simulink model "Wind_Turbine"  (R2018a)
settings: Solver=ode3  StartTime=0.0  StopTime=80  FixedStep=1e-4  RelTol=1e-3  EnableMultiTasking=on
InitFcn:
  | clear all ;
  | clc;
  | %Turbine
  | R_=45;
  | G=100;
  | lambda_opt=7.07;
  | Rho=1.225;
  | J=254;
  | f=0.01;
  | 
  | %RL filter;
  | 
  | fs=10000;
  | fe=50;
  | Ws=2*pi*fe;
  | Pres=3e6;
  | L=0.75e-3;
  | R=0.075;
  | c=38e-3;
  | 
  | %Commande CCR;
  | 
  | Id_=300;
  | Vdc_=1200;
  | %Vq_=0;
  | tr=0.001;
  | kp=3*L/tr;
  | ki=3*R/tr;
  | 
  | %CCM Commande;
  | 
  | p=2;p=2;
  | Tr=0.02;
  | Lfs=121e-6;
  | Lfr=57.3e-6;
  | Lm=12.12e-3;
  | m=1;
  | Ls=Lfs+Lm;
  | Lr=Lfr+m*Lm;
  | sigma=1-(m*Lm)^2/(Ls*Lr);
  | Rr=3.82e-3;
  | Rs=2.97e-3;
  | kpr=3*sigma*Lr/Tr;
  | kir=3*Rr/Tr;
  | Qs_ref=0;
undefined symbols (not defined in the file): sigbuilder_block
libraries: powerlib_meascontrol x8, simulink x4
settings Model: Creator=PC  LastModifiedBy=yassine
settings OptimizationCC: LifeSpan=inf
settings DebuggingCC: SFUnexpectedBacktrackingDiag=warning  SFNoUnconditionalDefaultTransitionDiag=warning
settings CodeAppCC: StateflowObjectComments=on
settings GRTTargetCC: TargetLangStandard=C89/C90 (ANSI)
settings ConfigComp: CovMetricSettings=dw  CovSaveCumulativeToWorkspaceVar=on  CovSaveSingleToWorkspaceVar=on  CovExternalEMLEnable=off

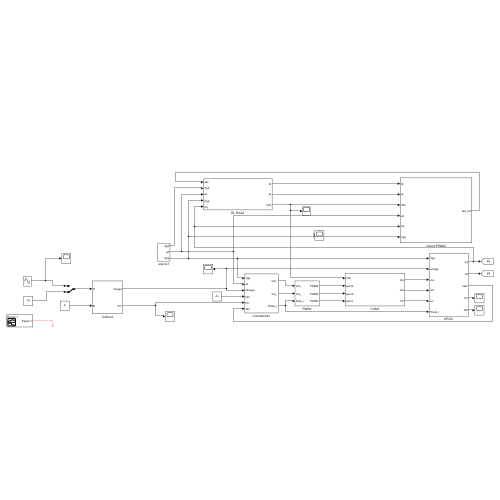
[thumbnail: Simulink's stored preview of the top-level diagram]
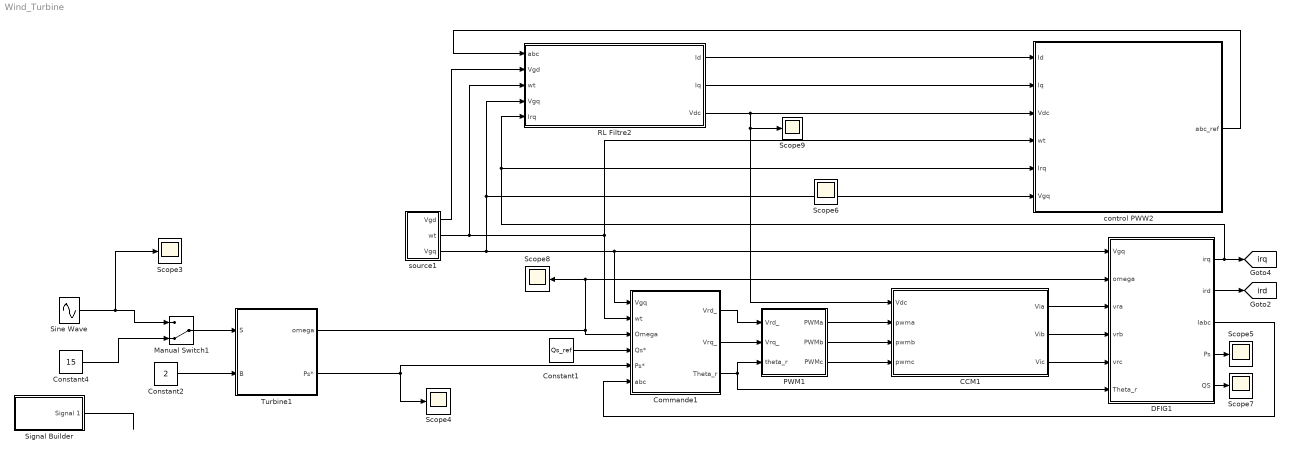
== system Wind_Turbine ==
  CCM1 : Subsystem
  Commande1 : Subsystem
  Constant1 : Constant  Value=Qs_ref
  Constant2 : Constant  Value=2
  Constant4 : Constant  Value=15
  DFIG1 : Subsystem
  Manual Switch1 : ManualSwitch  CurrentSetting=0
  PWM1 : Subsystem
  RL Filtre2 : Subsystem  InitFcn=""
  Scope{3..9} (7 alike) : Scope
  Signal Builder : Subsystem  Tag=STV Subsys  LoadFcn=sigbuilder_block('load');  StartFcn=sigbuilder_block('start');  StopFcn=sigbuilder_block('stop');  ClipboardFcn=sigbuilder_block('clipboard');  mask(Sigbuilder block){tuvar=[0:10]}
      mask help: Simulink:masks:SigbuilderBlock_MD
      mask init:
      | if ~strcmp(get_param(bdroot(gcbh),'SimulationStatus'),'stopped') tuvar = sigbuilder_block('maskInit'); end
      settings: CopyFcn=sigbuilder_block('copy');  DeleteFcn=sigbuilder_block('delete');  ModelCloseFcn=sigbuilder_block('modelClose');  PreSaveFcn=sigbuilder_block('preSave');  PauseFcn=sigbuilder_block('pause');  ContinueFcn=sigbuilder_block('continue');  NameChangeFcn=sigbuilder_block('namechange');  OpenFcn=sigbuilder_block('open',[525.6 43.2 550.8 400.2 ]);  CloseFcn=sigbuilder_block('close');
      mask Display: plot(0, 0, 100, 100,[2, 2, 32, 32, 2], [68, 8, 8, 68, 68],[32, 2], [38, 38], [32, 19, 2],[53, 60, 44], [32, 17, 17, 2],[16, 16, 31, 31]);txt = getActiveGroup(gcbh);text(2, 100, txt,'verticalAlignment', 'top');
  Sine Wave : Sin  Bias=9  Frequency=2*pi*1/80  SampleTime=0
  Turbine1 : Subsystem
  control PWW2 : Subsystem
  source1 : Subsystem
  tag scope: ird=global, irq=global
  wires:
  source1/2(wt) -> Commande1/2(wt), control PWW2/4(wt), RL Filtre2/3(wt)
  CCM1/1(Via) -> DFIG1/3(vra)
  CCM1/2(Vib) -> DFIG1/4(vrb)
  CCM1/3(Vic) -> DFIG1/5(vrc)
  RL Filtre2/3(Vdc) -> CCM1/1(Vdc), Scope9/1, control PWW2/3(Vdc)
  PWM1/2(PWMb) -> CCM1/3(pwmb)
  Commande1/1(Vrd_) -> PWM1/1(Vrd_)
  Commande1/2(Vrq_) -> PWM1/2(Vrq_)
  PWM1/1(PWMa) -> CCM1/2(pwma)
  PWM1/3(PWMc) -> CCM1/4(pwmc)
  source1/3(Vgq) -> Commande1/1(Vgq), DFIG1/1(Vgq), control PWW2/6(Vgq), RL Filtre2/4(Vgq)
  Commande1/3(Theta_r) -> DFIG1/6(Theta_r), PWM1/3(theta_r)
  DFIG1/3(Iabc) -> Commande1/6(abc)
  DFIG1/2(ird) -> [ird]
  Turbine1/1(omega) -> Scope8/1, DFIG1/2(omega), Commande1/3(Omega)
  DFIG1/4(Ps) -> Scope5/1
  DFIG1/5(QS) -> Scope7/1
  control PWW2/1(abc_ref) -> RL Filtre2/1(abc)
  RL Filtre2/1(Id) -> control PWW2/1(Id)
  RL Filtre2/2(Iq) -> control PWW2/2(Iq)
  DFIG1/1(irq) -> [irq], RL Filtre2/5(Irq), control PWW2/5(Irq)
  source1/1(Vgd) -> RL Filtre2/2(Vgd)
  Constant1/1 -> Commande1/4(Qs*)
  Turbine1/2(Ps*) -> Commande1/5(Ps*), Scope4/1
  Constant2/1 -> Turbine1/2(B)
  Sine Wave/1 -> Manual Switch1/1, Scope3/1
  Manual Switch1/1 -> Turbine1/1(S)
  Signal Builder/1(Signal 1) -> ?
  Constant4/1 -> Manual Switch1/2

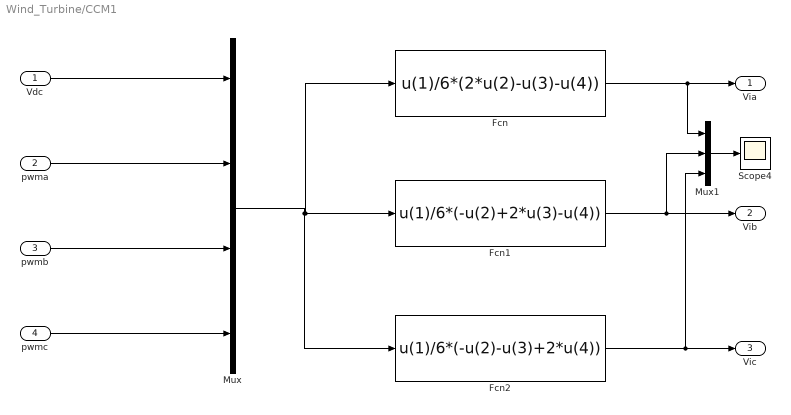
== system Wind_Turbine/CCM1 ==
  Vdc : Inport
  pwma : Inport  Port=2
  pwmb : Inport  Port=3
  pwmc : Inport  Port=4
  Fcn : Fcn  Expr=u(1)/6*(2*u(2)-u(3)-u(4))
  Fcn1 : Fcn  Expr=u(1)/6*(-u(2)+2*u(3)-u(4))
  Fcn2 : Fcn  Expr=u(1)/6*(-u(2)-u(3)+2*u(4))
  Mux : Mux
  Mux1 : Mux  Inputs=3
  Scope4 : Scope
  Via : Outport
  Vib : Outport  Port=2
  Vic : Outport  Port=3
  wires:
  Vdc/1 -> Mux/1
  Mux/1 -> Fcn2/1, Fcn1/1, Fcn/1
  pwma/1 -> Mux/2
  pwmb/1 -> Mux/3
  pwmc/1 -> Mux/4
  Fcn/1 -> Mux1/1, Via/1
  Fcn1/1 -> Vib/1, Mux1/2
  Fcn2/1 -> Vic/1, Mux1/3
  Mux1/1 -> Scope4/1

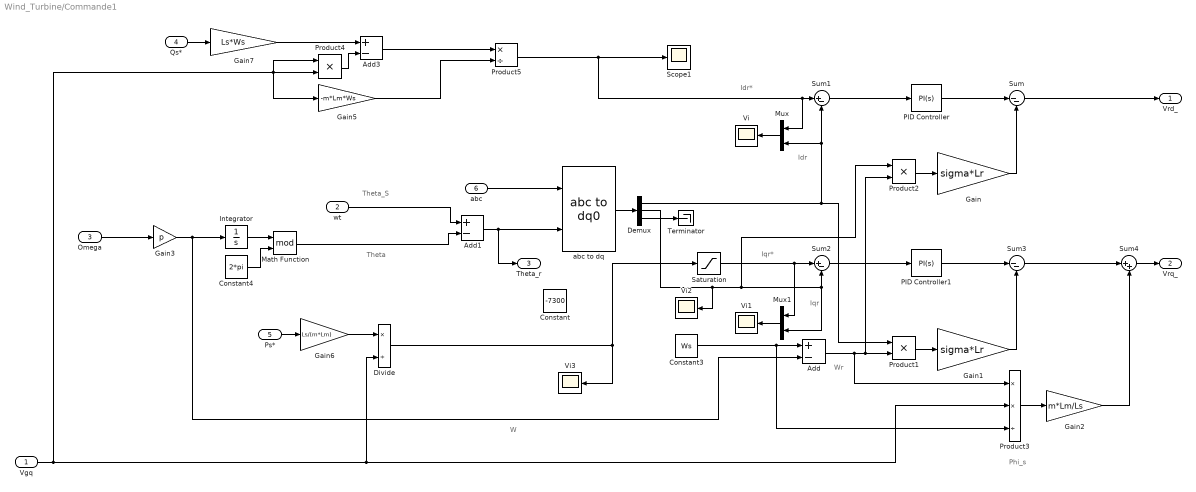
== system Wind_Turbine/Commande1 ==
  note: Theta_S
  note: Theta
  note: W
  note: Wr
  note: Iqr
  note: Idr
  note: Phi_s
  note: Idr*
  note: Iqr*
  Vgq : Inport
  wt : Inport  Port=2
  Omega : Inport  Port=3
  Qs* : Inport  Port=4
  Ps* : Inport  Port=5
  abc : Inport  Port=6
  Add : Sum  Inputs=+-
  Add1 : Sum  Inputs=+-
  Add3 : Sum  Inputs=+-
  Constant : Constant  Value=-7300
  Constant3 : Constant  Value=Ws
  Constant4 : Constant  Value=2*pi
  Demux : Demux  Outputs=3
  Divide : Product  Inputs=*/
  Gain : Gain  Gain=sigma*Lr
  Gain1 : Gain  Gain=sigma*Lr
  Gain2 : Gain  Gain=m*Lm/Ls
  Gain3 : Gain  Gain=p
  Gain5 : Gain  Gain=-m*Lm*Ws
  Gain6 : Gain  Gain=Ls/(m*Lm)
  Gain7 : Gain  Gain=Ls*Ws
  Integrator : Integrator
  Math Function : Math  Operator=mod  SaturateOnIntegerOverflow=on
  Mux : Mux  Inputs=2
  Mux1 : Mux  Inputs=2
  PID Controller : simulink/Continuous/PID Controller  Controller=PI  Form=Parallel  TimeDomain=Continuous-time  SampleTime=-1  IntegratorMethod=Forward Euler  ControllerParametersSource=internal  P=kpr*62  I=kir*62  D=0  N=100  UseFilter=on  TunerSelectOption=Transfer Function Based (PID Tuner App)  InitialConditionSource=internal  InitialConditionForIntegrator=0  InitialConditionForFilter=0  DifferentiatorICPrevScaledInput=0  ExternalReset=none  TrackingMode=off  Kt=1  LimitOutput=off  UpperSaturationLimit=inf  LowerSaturationLimit=-inf  LinearizeAsGain=on  AntiWindupMode=none  Kb=1  POutMin=[]  POutMax=[]  IOutMin=[]  IOutMax=[]  DOutMin=[]  DOutMax=[]  NOutMin=[]  NOutMax=[]  SumOutMin=[]  SumOutMax=[]  SaturationOutMin=[]  SaturationOutMax=[]  PParamMin=[]  PParamMax=[]  IParamMin=[]  IParamMax=[]  DParamMin=[]  DParamMax=[]  NParamMin=[]  NParamMax=[]  KbParamMin=[]  KbParamMax=[]  KtParamMin=[]  KtParamMax=[]  KbOutMin=[]  KbOutMax=[]  KtOutMin=[]  KtOutMax=[]  IntegratorOutMin=[]  IntegratorOutMax=[]  FilterOutMin=[]  FilterOutMax=[]  SumI1OutMin=[]  SumI1OutMax=[]  SumI2OutMin=[]  SumI2OutMax=[]  SumI3OutMin=[]  SumI3OutMax=[]  SumDOutMin=[]  SumDOutMax=[]  DifferentiatorOutMin=[]  DifferentiatorOutMax=[]  FilterDiffOutCoefMin=[]  FilterDiffOutCoefMax=[]  ReciprocalOutMin=[]  ReciprocalOutMax=[]  SumDenOutMin=[]  SumDenOutMax=[]  SumNumOutMin=[]  SumNumOutMax=[]  DivideOutMin=[]  DivideOutMax=[]  IntegratorContinuousStateAttributes=''  IntegratorStateMustResolveToSignalObject=off  IntegratorRTWStateStorageClass=Auto  FilterContinuousStateAttributes=''  FilterStateMustResolveToSignalObject=off  FilterRTWStateStorageClass=Auto
  PID Controller1 : simulink/Continuous/PID Controller  Controller=PI  Form=Parallel  TimeDomain=Continuous-time  SampleTime=-1  IntegratorMethod=Forward Euler  ControllerParametersSource=internal  P=kpr*62  I=kir*62  D=0  N=100  UseFilter=on  TunerSelectOption=Transfer Function Based (PID Tuner App)  InitialConditionSource=internal  InitialConditionForIntegrator=0  InitialConditionForFilter=0  DifferentiatorICPrevScaledInput=0  ExternalReset=none  TrackingMode=off  Kt=1  LimitOutput=off  UpperSaturationLimit=inf  LowerSaturationLimit=-inf  LinearizeAsGain=on  AntiWindupMode=none  Kb=1  POutMin=[]  POutMax=[]  IOutMin=[]  IOutMax=[]  DOutMin=[]  DOutMax=[]  NOutMin=[]  NOutMax=[]  SumOutMin=[]  SumOutMax=[]  SaturationOutMin=[]  SaturationOutMax=[]  PParamMin=[]  PParamMax=[]  IParamMin=[]  IParamMax=[]  DParamMin=[]  DParamMax=[]  NParamMin=[]  NParamMax=[]  KbParamMin=[]  KbParamMax=[]  KtParamMin=[]  KtParamMax=[]  KbOutMin=[]  KbOutMax=[]  KtOutMin=[]  KtOutMax=[]  IntegratorOutMin=[]  IntegratorOutMax=[]  FilterOutMin=[]  FilterOutMax=[]  SumI1OutMin=[]  SumI1OutMax=[]  SumI2OutMin=[]  SumI2OutMax=[]  SumI3OutMin=[]  SumI3OutMax=[]  SumDOutMin=[]  SumDOutMax=[]  DifferentiatorOutMin=[]  DifferentiatorOutMax=[]  FilterDiffOutCoefMin=[]  FilterDiffOutCoefMax=[]  ReciprocalOutMin=[]  ReciprocalOutMax=[]  SumDenOutMin=[]  SumDenOutMax=[]  SumNumOutMin=[]  SumNumOutMax=[]  DivideOutMin=[]  DivideOutMax=[]  IntegratorContinuousStateAttributes=''  IntegratorStateMustResolveToSignalObject=off  IntegratorRTWStateStorageClass=Auto  FilterContinuousStateAttributes=''  FilterStateMustResolveToSignalObject=off  FilterRTWStateStorageClass=Auto
  Product1 : Product
  Product2 : Product
  Product3 : Product  Inputs=**/
  Product4 : Product  Inputs=**
  Product5 : Product  Inputs=*/
  Saturation : Saturate  UpperLimit=8e3  LowerLimit=-8e3
  Scope1 : Scope
  Sum : Sum  Inputs=|--
  Sum1 : Sum  Inputs=|+-
  Sum2 : Sum  Inputs=|+-
  Sum3 : Sum  Inputs=|--
  Sum4 : Sum  Inputs=|++
  Terminator : Terminator
  Vi{,1..3} (4 alike) : Scope
  abc to dq : powerlib_meascontrol/Transformations/abc to dq0  Alignment=90 degrees behind phase A axis
  Vrd_ : Outport
  Vrq_ : Outport  Port=2
  Theta_r : Outport  Port=3
  wires:
  Sum2/1 -> PID Controller1/1
  Sum1/1 -> PID Controller/1
  Demux/2 -> Vi2/1, Mux1/2, Sum2/2, Product2/1
  PID Controller/1 -> Sum/1
  Gain/1 -> Sum/2
  Sum4/1 -> Vrq_/1
  PID Controller1/1 -> Sum3/1
  Demux/1 -> Sum1/2, Mux/2, Product1/1
  Gain2/1 -> Sum4/2
  Sum3/1 -> Sum4/1
  Sum/1 -> Vrd_/1
  Gain1/1 -> Sum3/2
  Constant3/1 -> Product3/3, Add/1
  Product1/1 -> Gain1/1
  Add/1 -> Product3/1, Product2/2, Product1/2
  Omega/1 -> Gain3/1
  Product2/1 -> Gain/1
  Product3/1 -> Gain2/1
  abc to dq/1 -> Demux/1
  Demux/3 -> Terminator/1
  abc/1 -> abc to dq/1
  wt/1 -> Add1/1
  Integrator/1 -> Math Function/1
  Constant4/1 -> Math Function/2
  Math Function/1 -> Add1/2
  Gain3/1 -> Integrator/1, Add/2
  Mux/1 -> Vi/1
  Mux1/1 -> Vi1/1
  Add1/1 -> abc to dq/2, Theta_r/1
  Add3/1 -> Product5/1
  Vgq/1 -> Product3/2, Divide/2, Product4/1, Gain5/1, Product4/2
  Qs*/1 -> Gain7/1
  Gain5/1 -> Product5/2
  Product5/1 -> Sum1/1, Mux/1, Scope1/1
  Ps*/1 -> Gain6/1
  Gain6/1 -> Divide/1
  Gain7/1 -> Add3/1
  Product4/1 -> Add3/2
  Divide/1 -> Vi3/1, Saturation/1
  Saturation/1 -> Mux1/1, Sum2/1

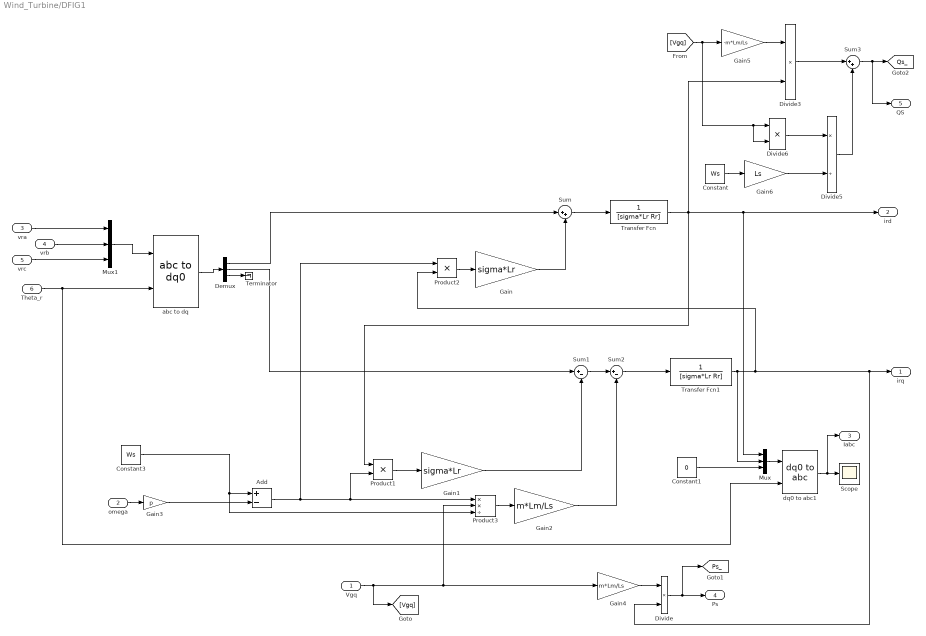
== system Wind_Turbine/DFIG1 ==
  Vgq : Inport
  omega : Inport  Port=2
  vra : Inport  Port=3
  vrb : Inport  Port=4
  vrc : Inport  Port=5
  Theta_r : Inport  Port=6
  Add : Sum  Inputs=+-
  Constant : Constant  Value=Ws
  Constant1 : Constant  Value=0
  Constant3 : Constant  Value=Ws
  Demux : Demux  Outputs=3
  Divide : Product  Inputs=**
  Divide3 : Product  Inputs=**
  Divide5 : Product  Inputs=*/
  Divide6 : Product  Inputs=**
  Gain : Gain  Gain=sigma*Lr
  Gain1 : Gain  Gain=sigma*Lr
  Gain2 : Gain  Gain=m*Lm/Ls
  Gain3 : Gain  Gain=p
  Gain4 : Gain  Gain=m*Lm/Ls
  Gain5 : Gain  Gain=-m*Lm/Ls
  Gain6 : Gain  Gain=Ls
  Mux : Mux  Inputs=3
  Mux1 : Mux  Inputs=3
  Product1 : Product
  Product2 : Product
  Product3 : Product  Inputs=**/
  Scope : Scope
  Sum : Sum  Inputs=|++
  Sum1 : Sum  Inputs=|+-
  Sum2 : Sum  Inputs=|+-
  Sum3 : Sum  Inputs=|++
  Terminator : Terminator
  Transfer Fcn : TransferFcn  Denominator=[sigma*Lr Rr]
  Transfer Fcn1 : TransferFcn  Denominator=[sigma*Lr Rr]
  abc to dq : powerlib_meascontrol/Transformations/abc to dq0  Alignment=90 degrees behind phase A axis
  dq0 to abc1 : powerlib_meascontrol/Transformations/dq0 to abc  Alignment=90 degrees behind phase A axis
  irq : Outport
  ird : Outport  Port=2
  Iabc : Outport  Port=3
  Ps : Outport  Port=4
  QS : Outport  Port=5
  tag scope: Ps_=global, Qs_=global
  wires:
  Transfer Fcn/1 -> ird/1, Mux/1, Divide3/2, Product1/1
  Sum/1 -> Transfer Fcn/1
  Demux/2 -> Sum1/1
  Demux/1 -> Sum/1
  Product2/1 -> Gain/1
  Gain/1 -> Sum/2
  Constant3/1 -> Product3/3, Add/1
  Product1/1 -> Gain1/1
  Product3/1 -> Gain2/1
  Sum1/1 -> Sum2/1
  Gain1/1 -> Sum1/2
  Gain2/1 -> Sum2/2
  Sum2/1 -> Transfer Fcn1/1
  Add/1 -> Product2/1, Product1/2, Product3/1
  omega/1 -> Gain3/1
  Gain3/1 -> Add/2
  Constant1/1 -> Mux/3
  Mux/1 -> dq0 to abc1/1
  dq0 to abc1/1 -> Iabc/1, Scope/1
  abc to dq/1 -> Demux/1
  Demux/3 -> Terminator/1
  Mux1/1 -> abc to dq/1
  vra/1 -> Mux1/1
  vrb/1 -> Mux1/2
  vrc/1 -> Mux1/3
  Theta_r/1 -> dq0 to abc1/2, abc to dq/2
  Transfer Fcn1/1 -> irq/1, Divide/2, Product2/2, Mux/2
  Divide/1 -> Ps/1, [Ps_]
  Gain4/1 -> Divide/1
  Gain5/1 -> Divide3/1
  Divide3/1 -> Sum3/1
  Sum3/1 -> QS/1, [Qs_]
  [Vgq] -> Divide6/2, Divide6/1, Gain5/1
  Divide6/1 -> Divide5/1
  Gain6/1 -> Divide5/2
  Constant/1 -> Gain6/1
  Divide5/1 -> Sum3/2
  Vgq/1 -> [Vgq], Product3/2, Gain4/1

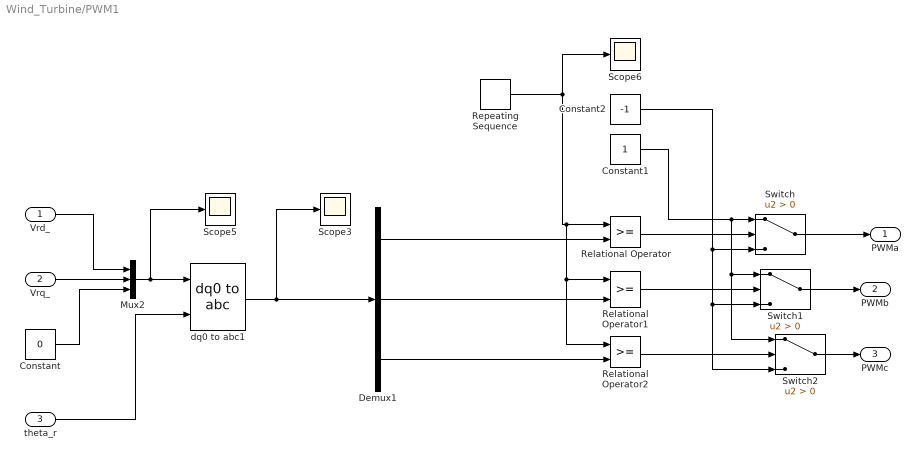
== system Wind_Turbine/PWM1 ==
  Vrd_ : Inport
  Vrq_ : Inport  Port=2
  theta_r : Inport  Port=3
  Constant : Constant  Value=0
  Constant1 : Constant
  Constant2 : Constant  Value=-1
  Demux1 : Demux  Outputs=3
  Mux2 : Mux  Inputs=3
  Relational Operator : RelationalOperator  OutDataTypeStr=boolean  RndMeth=Nearest
  Relational Operator1 : RelationalOperator  OutDataTypeStr=boolean  RndMeth=Nearest
  Relational Operator2 : RelationalOperator  OutDataTypeStr=boolean  RndMeth=Nearest
  Repeating Sequence : simulink/Sources/Repeating Sequence  rep_seq_t=[0 1/40000 1/20000 3/40000 1/10000]  rep_seq_y="[0 600  0 -600 0]"
  Scope3 : Scope
  Scope5 : Scope
  Scope6 : Scope
  Switch : Switch  Criteria=u2 > Threshold
  Switch1 : Switch  Criteria=u2 > Threshold
  Switch2 : Switch  Criteria=u2 > Threshold
  dq0 to abc1 : powerlib_meascontrol/Transformations/dq0 to abc  Alignment=90 degrees behind phase A axis
  PWMa : Outport
  PWMb : Outport  Port=2
  PWMc : Outport  Port=3
  wires:
  Constant/1 -> Mux2/3
  Switch2/1 -> PWMc/1
  Switch1/1 -> PWMb/1
  Switch/1 -> PWMa/1
  Demux1/2 -> Relational Operator1/2
  Demux1/3 -> Relational Operator2/2
  Demux1/1 -> Relational Operator/2
  Repeating Sequence/1 -> Scope6/1, Relational Operator2/1, Relational Operator1/1, Relational Operator/1
  Constant2/1 -> Switch/3, Switch1/3, Switch2/3
  Mux2/1 -> dq0 to abc1/1, Scope5/1
  Relational Operator2/1 -> Switch2/2
  Vrd_/1 -> Mux2/1
  Constant1/1 -> Switch1/1, Switch2/1, Switch/1
  Relational Operator/1 -> Switch/2
  Relational Operator1/1 -> Switch1/2
  Vrq_/1 -> Mux2/2
  theta_r/1 -> dq0 to abc1/2
  dq0 to abc1/1 -> Demux1/1, Scope3/1

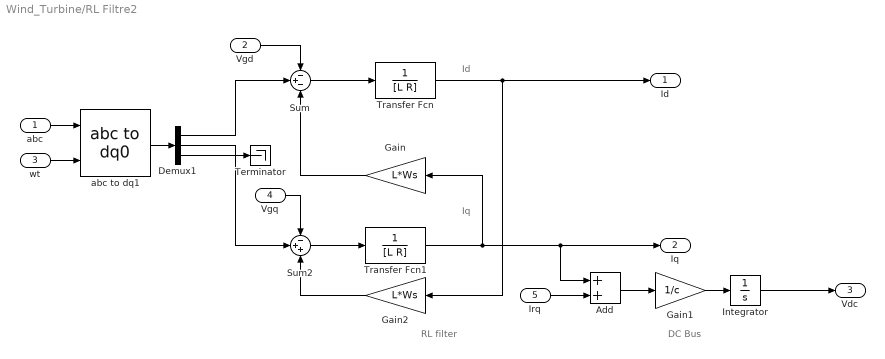
== system Wind_Turbine/RL Filtre2 ==
  note: RL filter
  note: DC Bus
  note: Id
  note: Iq
  abc : Inport
  Vgd : Inport  Port=2
  wt : Inport  Port=3
  Vgq : Inport  Port=4
  Irq : Inport  Port=5
  Add : Sum
  Demux1 : Demux  Outputs=3
  Gain : Gain  Gain=L*Ws
  Gain1 : Gain  Gain=1/c
  Gain2 : Gain  Gain=L*Ws
  Integrator : Integrator  UpperSaturationLimit=2000  LowerSaturationLimit=-2000
  Sum : Sum  Inputs=-+-
  Sum2 : Sum  Inputs=-++
  Terminator : Terminator
  Transfer Fcn : TransferFcn  Denominator=[L R]
  Transfer Fcn1 : TransferFcn  Denominator=[L R]
  abc to dq1 : powerlib_meascontrol/Transformations/abc to dq0  Alignment=90 degrees behind phase A axis
  Id : Outport
  Iq : Outport  Port=2
  Vdc : Outport  Port=3
  wires:
  Transfer Fcn1/1 -> Iq/1, Add/1, Gain/1
  abc to dq1/1 -> Demux1/1
  Demux1/3 -> Terminator/1
  abc/1 -> abc to dq1/1
  wt/1 -> abc to dq1/2
  Sum/1 -> Transfer Fcn/1
  Sum2/1 -> Transfer Fcn1/1
  Gain/1 -> Sum/3
  Gain2/1 -> Sum2/3
  Add/1 -> Gain1/1
  Gain1/1 -> Integrator/1
  Transfer Fcn/1 -> Id/1, Gain2/1
  Demux1/2 -> Sum2/2
  Demux1/1 -> Sum/2
  Irq/1 -> Add/2
  Vgq/1 -> Sum2/1
  Vgd/1 -> Sum/1
  Integrator/1 -> Vdc/1

== system Wind_Turbine/Signal Builder ==
  Demux : Demux  Tag=STV Demux  Outputs=1
      settings: DisplayOption=none
  FromWs : FromWorkspace  Tag=STV FromWs  VariableName=tuvar
      SigBuilderData=|
      | common.afterFinalStr = 'Extrapolate'
      | common.sampleTime = 0
      | dataSet.timeRange = [0 10]
      | dataSet.name = 'Group 1'
      | sbobj.Groups.Name = 'Group 1'
      | sbobj.Groups.Signals.Name = 'Signal 1'
      | sbobj.Groups.Signals.XData = [0 1 2 3 4 5 6 7 8 9 10]
      | sbobj.Groups.Signals.YData = [5 4 6 8.6 8.65 8.75 5.95 0.65 2 0.65 0.7]
  Signal 1 : Outport  Tag=STV Outport
  wires:
  FromWs/1 -> Demux/1
  Demux/1 -> Signal 1/1

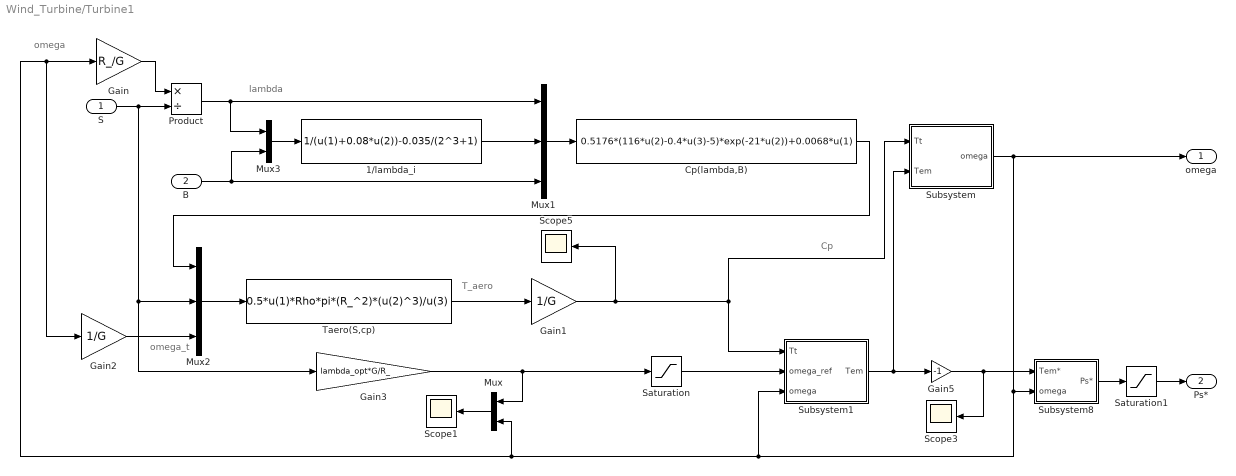
== system Wind_Turbine/Turbine1 ==
  note: T_aero
  note: omega_t
  note: omega
  note: lambda
  note: Cp
  S : Inport
  B : Inport  Port=2
  1/lambda_i : Fcn  Expr=1/(u(1)+0.08*u(2))-0.035/(2^3+1)
  Cp(lambda,B) : Fcn  Expr=0.5176*(116*u(2)-0.4*u(3)-5)*exp(-21*u(2))+0.0068*u(1)
  Gain : Gain  Gain=R_/G
  Gain1 : Gain  Gain=1/G
  Gain2 : Gain  Gain=1/G
  Gain3 : Gain  Gain=lambda_opt*G/R_
  Gain5 : Gain  Gain=-1
  Mux : Mux  Inputs=2
  Mux1 : Mux  Inputs=3
  Mux2 : Mux  Inputs=3
  Mux3 : Mux  Inputs=2
  Product : Product  Inputs=*/
  Saturation : Saturate  UpperLimit=200  LowerLimit=60
  Saturation1 : Saturate  UpperLimit=0  LowerLimit=-3e6
  Scope1 : Scope
  Scope3 : Scope
  Scope5 : Scope
  Subsystem : Subsystem
  Subsystem1 : Subsystem
  Subsystem8 : Subsystem
  Taero(S,cp) : Fcn  Expr=0.5*u(1)*Rho*pi*(R_^2)*(u(2)^3)/u(3)
  omega : Outport
  Ps* : Outport  Port=2
  wires:
  Subsystem8/1(Ps*) -> Saturation1/1
  1/lambda_i/1 -> Mux1/2
  B/1 -> Mux1/3, Mux3/2
  Product/1 -> Mux3/1, Mux1/1
  S/1 -> Gain3/1, Mux2/2, Product/2
  Cp(lambda,B)/1 -> Mux2/1
  Gain/1 -> Product/1
  Gain2/1 -> Mux2/3
  Mux1/1 -> Cp(lambda,B)/1
  Mux2/1 -> Taero(S,cp)/1
  Taero(S,cp)/1 -> Gain1/1
  Mux/1 -> Scope1/1
  Mux3/1 -> 1/lambda_i/1
  Gain5/1 -> Subsystem8/1(Tem*), Scope3/1
  Subsystem1/1(Tem) -> Subsystem/2(Tem), Gain5/1
  Subsystem/1(omega) -> omega/1, Gain/1, Gain2/1, Mux/2, Subsystem1/3(omega), Subsystem8/2(omega)
  Gain1/1 -> Scope5/1, Subsystem1/1(Tt), Subsystem/1(Tt)
  Gain3/1 -> Saturation/1, Mux/1
  Saturation/1 -> Subsystem1/2(omega_ref)
  Saturation1/1 -> Ps*/1

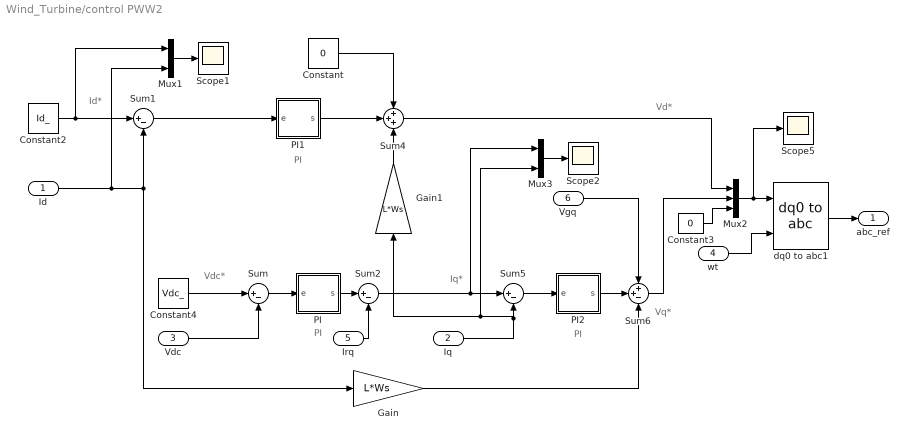
== system Wind_Turbine/control PWW2 ==
  note: PI
  note: Iq*
  note: Vq*
  note: Vd*
  note: Id*
  note: Vdc*
  note: PI
  note: PI
  Id : Inport
  Iq : Inport  Port=2
  Vdc : Inport  Port=3
  wt : Inport  Port=4
  Irq : Inport  Port=5
  Vgq : Inport  Port=6
  Constant : Constant  Value=0
  Constant2 : Constant  Value=Id_
  Constant3 : Constant  Value=0
  Constant4 : Constant  Value=Vdc_
  Gain : Gain  Gain=L*Ws
  Gain1 : Gain  Gain=L*Ws
  Mux1 : Mux  Inputs=2
  Mux2 : Mux  Inputs=3
  Mux3 : Mux  Inputs=2
  PI : Subsystem
  PI1 : Subsystem
  PI2 : Subsystem
  Scope1 : Scope
  Scope2 : Scope
  Scope5 : Scope
  Sum{,1..2,5} (4 alike) : Sum  Inputs=|+-
  Sum4 : Sum  Inputs=+++
  Sum6 : Sum  Inputs=++-
  dq0 to abc1 : powerlib_meascontrol/Transformations/dq0 to abc  Alignment=90 degrees behind phase A axis
  abc_ref : Outport
  wires:
  Sum1/1 -> PI1/1(e)
  Vdc/1 -> Sum/2
  Sum/1 -> PI/1(e)
  PI/1(s) -> Sum2/1
  Constant2/1 -> Mux1/1, Sum1/1
  PI1/1(s) -> Sum4/2
  Constant3/1 -> Mux2/3
  Constant4/1 -> Sum/1
  Mux2/1 -> dq0 to abc1/1, Scope5/1
  dq0 to abc1/1 -> abc_ref/1
  wt/1 -> dq0 to abc1/2
  PI2/1(s) -> Sum6/2
  Id/1 -> Mux1/2, Sum1/2, Gain/1
  Sum6/1 -> Mux2/2
  Sum5/1 -> PI2/1(e)
  Sum4/1 -> Mux2/1
  Vgq/1 -> Sum6/1
  Gain/1 -> Sum6/3
  Irq/1 -> Sum2/2
  Constant/1 -> Sum4/1
  Gain1/1 -> Sum4/3
  Mux1/1 -> Scope1/1
  Sum2/1 -> Sum5/1, Mux3/1
  Iq/1 -> Sum5/2, Mux3/2, Gain1/1
  Mux3/1 -> Scope2/1

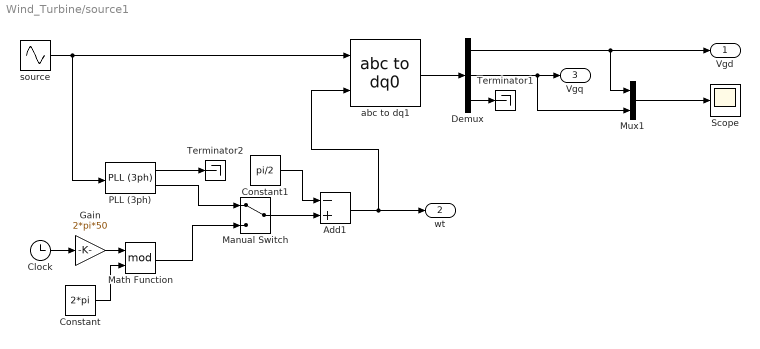
== system Wind_Turbine/source1 ==
  Add1 : Sum  Inputs=-+
  Clock : Clock
  Constant : Constant  Value=2*pi
  Constant1 : Constant  Value=pi/2
  Demux : Demux  Outputs=3
  Gain : Gain  Gain=2*pi*50
  Manual Switch : ManualSwitch
  Math Function : Math  Operator=mod  SaturateOnIntegerOverflow=on
  Mux1 : Mux  Inputs=2
  PLL (3ph) : powerlib_meascontrol/PLL/PLL (3ph)  Fmin=45  Par_Init=[0, 50]  ParK=[180, 3200, 1]  TcD=1e-4  MaxRateChangeFreq=12  FilterCutOffFreq=25  Ts=0  AGC=on
  Scope : Scope
  Terminator1 : Terminator
  Terminator2 : Terminator
  abc to dq1 : powerlib_meascontrol/Transformations/abc to dq0  Alignment=90 degrees behind phase A axis
  source : Sin  Amplitude=690*sqrt(2)/sqrt(3)  Frequency=2*pi*50  Phase=[0 -2*pi/3 2*pi/3]  SampleTime=0
  Vgd : Outport
  wt : Outport  Port=2
  Vgq : Outport  Port=3
  wires:
  abc to dq1/1 -> Demux/1
  source/1 -> abc to dq1/1, PLL (3ph)/1
  Demux/2 -> Mux1/2, Vgq/1
  Demux/3 -> Terminator1/1
  Demux/1 -> Mux1/1, Vgd/1
  PLL (3ph)/1 -> Terminator2/1
  Clock/1 -> Gain/1
  PLL (3ph)/2 -> Manual Switch/1
  Gain/1 -> Math Function/1
  Constant/1 -> Math Function/2
  Math Function/1 -> Manual Switch/2
  Add1/1 -> abc to dq1/2, wt/1
  Mux1/1 -> Scope/1
  Constant1/1 -> Add1/1
  Manual Switch/1 -> Add1/2

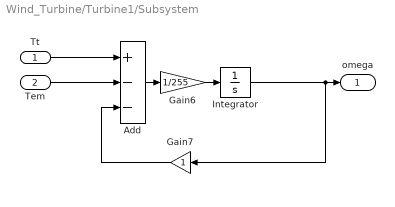
== system Wind_Turbine/Turbine1/Subsystem ==
  Tt : Inport
  Tem : Inport  Port=2
  Add : Sum  Inputs=+--
  Gain6 : Gain  Gain=1/255
  Gain7 : Gain
  Integrator : Integrator  InitialCondition=100  LowerSaturationLimit=1e-5
  omega : Outport
  wires:
  Add/1 -> Gain6/1
  Integrator/1 -> Gain7/1, omega/1
  Gain6/1 -> Integrator/1
  Tt/1 -> Add/1
  Gain7/1 -> Add/3
  Tem/1 -> Add/2

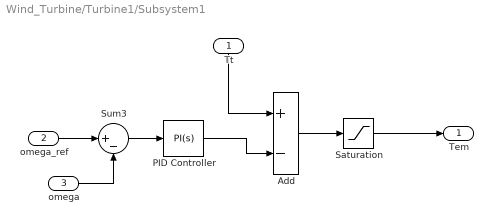
== system Wind_Turbine/Turbine1/Subsystem1 ==
  Tt : Inport
  omega_ref : Inport  Port=2
  omega : Inport  Port=3
  Add : Sum  Inputs=+-
  PID Controller : simulink/Continuous/PID Controller  Controller=PI  Form=Parallel  TimeDomain=Continuous-time  SampleTime=-1  IntegratorMethod=Forward Euler  ControllerParametersSource=internal  P=255  I=1  D=0  N=100  UseFilter=on  TunerSelectOption=Transfer Function Based (PID Tuner App)  InitialConditionSource=internal  InitialConditionForIntegrator=0  InitialConditionForFilter=0  DifferentiatorICPrevScaledInput=0  ExternalReset=none  TrackingMode=off  Kt=1  LimitOutput=off  UpperSaturationLimit=inf  LowerSaturationLimit=0  LinearizeAsGain=on  AntiWindupMode=none  Kb=1  POutMin=[]  POutMax=[]  IOutMin=[]  IOutMax=[]  DOutMin=[]  DOutMax=[]  NOutMin=[]  NOutMax=[]  SumOutMin=[]  SumOutMax=[]  SaturationOutMin=[]  SaturationOutMax=[]  PParamMin=[]  PParamMax=[]  IParamMin=[]  IParamMax=[]  DParamMin=[]  DParamMax=[]  NParamMin=[]  NParamMax=[]  KbParamMin=[]  KbParamMax=[]  KtParamMin=[]  KtParamMax=[]  KbOutMin=[]  KbOutMax=[]  KtOutMin=[]  KtOutMax=[]  IntegratorOutMin=[]  IntegratorOutMax=[]  FilterOutMin=[]  FilterOutMax=[]  SumI1OutMin=[]  SumI1OutMax=[]  SumI2OutMin=[]  SumI2OutMax=[]  SumI3OutMin=[]  SumI3OutMax=[]  SumDOutMin=[]  SumDOutMax=[]  DifferentiatorOutMin=[]  DifferentiatorOutMax=[]  FilterDiffOutCoefMin=[]  FilterDiffOutCoefMax=[]  ReciprocalOutMin=[]  ReciprocalOutMax=[]  SumDenOutMin=[]  SumDenOutMax=[]  SumNumOutMin=[]  SumNumOutMax=[]  DivideOutMin=[]  DivideOutMax=[]  IntegratorContinuousStateAttributes=''  IntegratorStateMustResolveToSignalObject=off  IntegratorRTWStateStorageClass=Auto  FilterContinuousStateAttributes=''  FilterStateMustResolveToSignalObject=off  FilterRTWStateStorageClass=Auto
  Saturation : Saturate  UpperLimit=1.9e4  LowerLimit=0
  Sum3 : Sum  Inputs=|+-
  Tem : Outport
  wires:
  Tt/1 -> Add/1
  Saturation/1 -> Tem/1
  Add/1 -> Saturation/1
  PID Controller/1 -> Add/2
  omega_ref/1 -> Sum3/1
  Sum3/1 -> PID Controller/1
  omega/1 -> Sum3/2

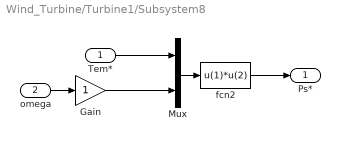
== system Wind_Turbine/Turbine1/Subsystem8 ==
  Tem* : Inport
  omega : Inport  Port=2
  Gain : Gain
  Mux : Mux  Inputs=2
  fcn2 : Fcn  Expr=u(1)*u(2)
  Ps* : Outport
  wires:
  Gain/1 -> Mux/2
  Tem*/1 -> Mux/1
  fcn2/1 -> Ps*/1
  omega/1 -> Gain/1
  Mux/1 -> fcn2/1

== system Wind_Turbine/control PWW2/PI ==
  e : Inport
  Add : Sum
  Gain : Gain  Gain=1.45
  Gain1 : Gain  Gain=27.27
  Integrator : Integrator  UpperSaturationLimit=350  LowerSaturationLimit=-350
  s : Outport
  wires:
  Gain/1 -> Add/1
  Gain1/1 -> Integrator/1
  Integrator/1 -> Add/2
  e/1 -> Gain/1, Gain1/1
  Add/1 -> s/1

== system Wind_Turbine/control PWW2/PI1 ==
  e : Inport
  Add : Sum
  Gain : Gain  Gain=kp
  Gain1 : Gain  Gain=ki
  Integrator : Integrator  UpperSaturationLimit=600  LowerSaturationLimit=-600
  s : Outport
  wires:
  Add/1 -> s/1
  e/1 -> Gain/1, Gain1/1
  Integrator/1 -> Add/2
  Gain1/1 -> Integrator/1
  Gain/1 -> Add/1

== system Wind_Turbine/control PWW2/PI2 ==
  e : Inport
  Add : Sum
  Gain : Gain  Gain=kp
  Gain1 : Gain  Gain=ki
  Integrator : Integrator  UpperSaturationLimit=600  LowerSaturationLimit=-600
  s : Outport
  wires:
  Add/1 -> s/1
  e/1 -> Gain/1, Gain1/1
  Integrator/1 -> Add/2
  Gain1/1 -> Integrator/1
  Gain/1 -> Add/1
